simulink model "model_0318"  (R2025b)
settings: Solver=ode4  StartTime=0.0  StopTime=10  FixedStep=1e-4  RelTol=1e-3
undefined symbols (not defined in the file or in its folder): dspblkCoreblockFVToolHelper, gcbh
libraries: simulink x9, dspfdesign x3, dspstat3 x2

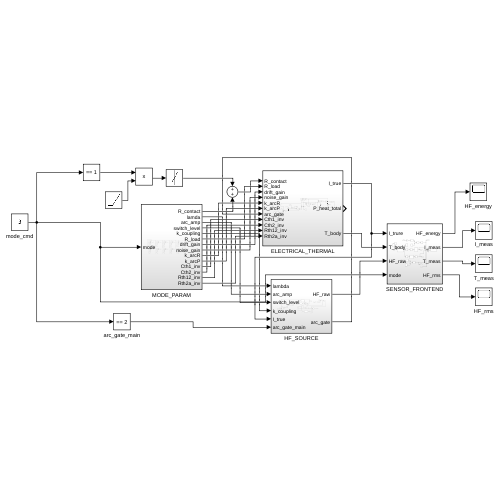
[thumbnail: Simulink's stored preview of the top-level diagram]
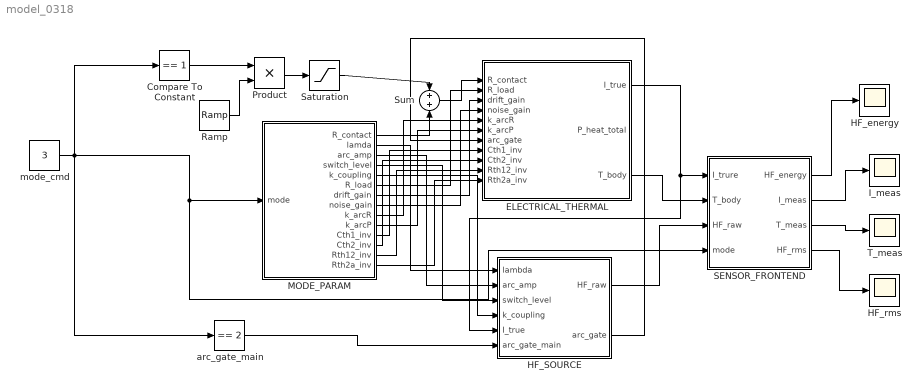
== system model_0318 ==
  Compare To Constant : simulink/Logic and Bit Operations/Compare To Constant  relop===  const=1  OutDataTypeStr=boolean
  ELECTRICAL_THERMAL : Subsystem
  HF_SOURCE : Subsystem
  HF_energy : Scope
      settings: ActiveDisplayYMinimum=-0.0012745703984799416  ActiveDisplayYMaximum=0.011471133695894987
  HF_rms : Scope
      settings: ActiveDisplayYMinimum=-0.0022642888342853068  ActiveDisplayYMaximum=0.020378601958750724  DataLoggingVariableName=ScopeData3
  I_meas : Scope
      settings: ActiveDisplayYMinimum=-209.09631630294618  ActiveDisplayYMaximum=207.20339945692962
  MODE_PARAM : Subsystem
  Product : Product
  Ramp : simulink/Sources/Ramp  slope=0.002  start=0  InitialOutput=0
  SENSOR_FRONTEND : Subsystem
  Saturation : Saturate  UpperLimit=0.05  LowerLimit=0
  Sum : Sum
  T_meas : Scope
      settings: ActiveDisplayYMinimum=19.005455597500632  ActiveDisplayYMaximum=28.950899622494315  DataLoggingVariableName=ScopeData2
  arc_gate_main : simulink/Logic and Bit Operations/Compare To Constant  relop===  const=2  OutDataTypeStr=boolean
  mode_cmd : Constant  Value=3
  wires:
  ELECTRICAL_THERMAL/1(I_true) -> HF_SOURCE/5(I_true), SENSOR_FRONTEND/1(I_trure)
  mode_cmd/1 -> arc_gate_main/1, SENSOR_FRONTEND/4(mode), MODE_PARAM/1(mode), Compare To Constant/1
  Compare To Constant/1 -> Product/1
  Ramp/1 -> Product/2
  Product/1 -> Saturation/1
  Saturation/1 -> Sum/1
  MODE_PARAM/1(R_contact) -> Sum/2
  Sum/1 -> ELECTRICAL_THERMAL/1(R_contact)
  SENSOR_FRONTEND/2(I_meas) -> I_meas/1
  SENSOR_FRONTEND/3(T_meas) -> T_meas/1
  SENSOR_FRONTEND/1(HF_energy) -> HF_energy/1
  SENSOR_FRONTEND/4(HF_rms) -> HF_rms/1
  MODE_PARAM/6(R_load) -> ELECTRICAL_THERMAL/2(R_load)
  MODE_PARAM/7(drift_gain) -> ELECTRICAL_THERMAL/3(drift_gain)
  MODE_PARAM/8(noise_gain) -> ELECTRICAL_THERMAL/4(noise_gain)
  MODE_PARAM/9(k_arcR) -> ELECTRICAL_THERMAL/5(k_arcR)
  MODE_PARAM/10(k_arcP) -> ELECTRICAL_THERMAL/6(k_arcP)
  MODE_PARAM/11(Cth1_inv) -> ELECTRICAL_THERMAL/8(Cth1_inv)
  MODE_PARAM/12(Cth2_inv) -> ELECTRICAL_THERMAL/9(Cth2_inv)
  MODE_PARAM/13(Rth12_inv) -> ELECTRICAL_THERMAL/10(Rth12_inv)
  MODE_PARAM/14(Rth2a_inv) -> ELECTRICAL_THERMAL/11(Rth2a_inv)
  MODE_PARAM/3(arc_amp) -> HF_SOURCE/2(arc_amp)
  MODE_PARAM/2(lamda) -> HF_SOURCE/1(lambda)
  MODE_PARAM/5(k_coupling) -> HF_SOURCE/4(k_coupling)
  MODE_PARAM/4(switch_level) -> HF_SOURCE/3(switch_level)
  HF_SOURCE/2(arc_gate) -> ELECTRICAL_THERMAL/7(arc_gate)
  HF_SOURCE/1(HF_raw) -> SENSOR_FRONTEND/3(HF_raw)
  ELECTRICAL_THERMAL/3(T_body) -> SENSOR_FRONTEND/2(T_body)
  arc_gate_main/1 -> HF_SOURCE/6(arc_gate_main)

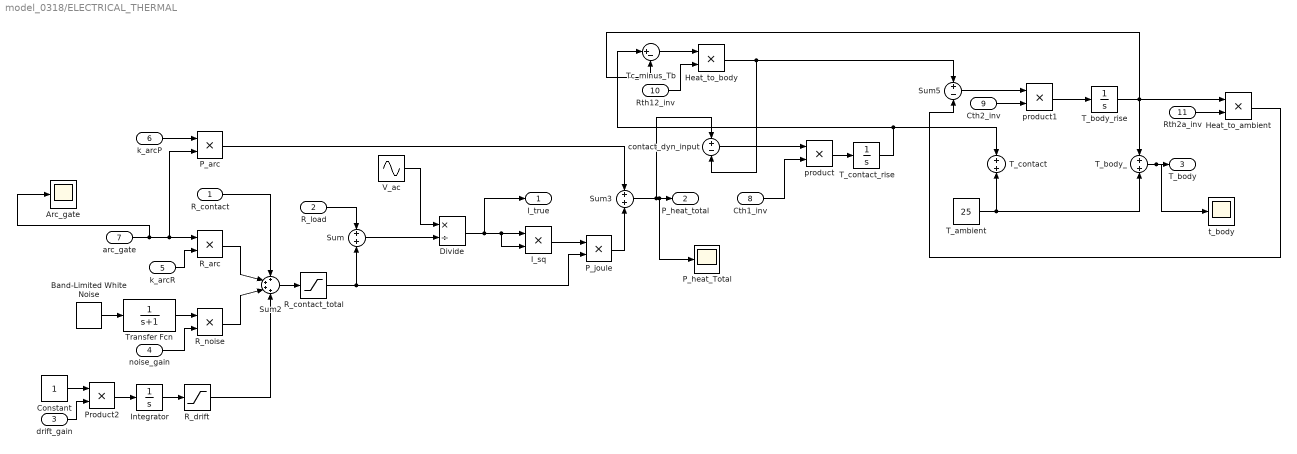
== system model_0318/ELECTRICAL_THERMAL ==
  R_contact : Inport
  R_load : Inport  Port=2
  drift_gain : Inport  Port=3
  noise_gain : Inport  Port=4
  k_arcR : Inport  Port=5
  k_arcP : Inport  Port=6
  arc_gate : Inport  Port=7
  Cth1_inv : Inport  Port=8
  Cth2_inv : Inport  Port=9
  Rth12_inv : Inport  Port=10
  Rth2a_inv : Inport  Port=11
  Arc_gate : Scope
      settings: ActiveDisplayYMinimum=-1  ActiveDisplayYMaximum=1  DataLoggingVariableName=ScopeData5
  Band-Limited White Noise : simulink/Sources/Band-Limited White Noise  Cov=1e-4  Ts=1e-4  seed=11
  Constant : Constant
  Divide : Product  Inputs=*/
  Heat_to_ambient : Product
  Heat_to_body : Product
  I_sq : Product
  Integrator : Integrator
  P_arc : Product
  P_heat_Total : Scope
      settings: ActiveDisplayYMinimum=-108.37902275446248  ActiveDisplayYMaximum=975.41120479016263  DataLoggingVariableName=ScopeData4
  P_joule : Product
  Product2 : Product
  R_arc : Product
  R_contact_total : Saturate  UpperLimit=1  LowerLimit=0.001
  R_drift : Saturate
  R_noise : Product
  Sum : Sum
  Sum2 : Sum  Inputs=++++
  Sum3 : Sum
  Sum5 : Sum  Inputs=+-
  T_ambient : Constant  Value=25
  T_body_ : Sum
  T_body_rise : Integrator
  T_contact : Sum
  T_contact_rise : Integrator
  Tc_minus_Tb : Sum  Inputs=|+-
  Transfer Fcn : TransferFcn  Denominator=[1 1]
  V_ac : Sin  Amplitude=311  Frequency=2*pi*60  SampleTime=1e-4
  contact_dyn_input : Sum  Inputs=+-
  product : Product
  product1 : Product
  t_body : Scope
      settings: ActiveDisplayYMinimum=14.417043129702609  ActiveDisplayYMaximum=120.24661183267655  DataLoggingVariableName=ScopeData7
  I_true : Outport
  P_heat_total : Outport  Port=2
  T_body : Outport  Port=3
  wires:
  R_load/1 -> Sum/1
  Sum/1 -> Divide/2
  V_ac/1 -> Divide/1
  Divide/1 -> I_sq/2, I_sq/1, I_true/1
  I_sq/1 -> P_joule/1
  P_joule/1 -> Sum3/2
  Band-Limited White Noise/1 -> Transfer Fcn/1
  Constant/1 -> Product2/1
  drift_gain/1 -> Product2/2
  Product2/1 -> Integrator/1
  Integrator/1 -> R_drift/1
  Transfer Fcn/1 -> R_noise/1
  noise_gain/1 -> R_noise/2
  arc_gate/1 -> Arc_gate/1, P_arc/2, R_arc/1
  k_arcR/1 -> R_arc/2
  R_contact/1 -> Sum2/1
  R_arc/1 -> Sum2/2
  R_noise/1 -> Sum2/3
  R_drift/1 -> Sum2/4
  Sum2/1 -> R_contact_total/1
  R_contact_total/1 -> P_joule/2, Sum/2
  k_arcP/1 -> P_arc/1
  P_arc/1 -> Sum3/1
  Sum3/1 -> contact_dyn_input/1, P_heat_Total/1, P_heat_total/1
  Tc_minus_Tb/1 -> Heat_to_body/1
  Heat_to_body/1 -> contact_dyn_input/2, Sum5/1
  Cth1_inv/1 -> product/2
  contact_dyn_input/1 -> product/1
  product/1 -> T_contact_rise/1
  T_contact_rise/1 -> T_contact/1, Tc_minus_Tb/1
  Sum5/1 -> product1/1
  Cth2_inv/1 -> product1/2
  product1/1 -> T_body_rise/1
  T_body_rise/1 -> T_body_/1, Heat_to_ambient/1, Tc_minus_Tb/2
  T_ambient/1 -> T_contact/2, T_body_/2
  Rth12_inv/1 -> Heat_to_body/2
  Rth2a_inv/1 -> Heat_to_ambient/2
  Heat_to_ambient/1 -> Sum5/2
  T_body_/1 -> t_body/1, T_body/1

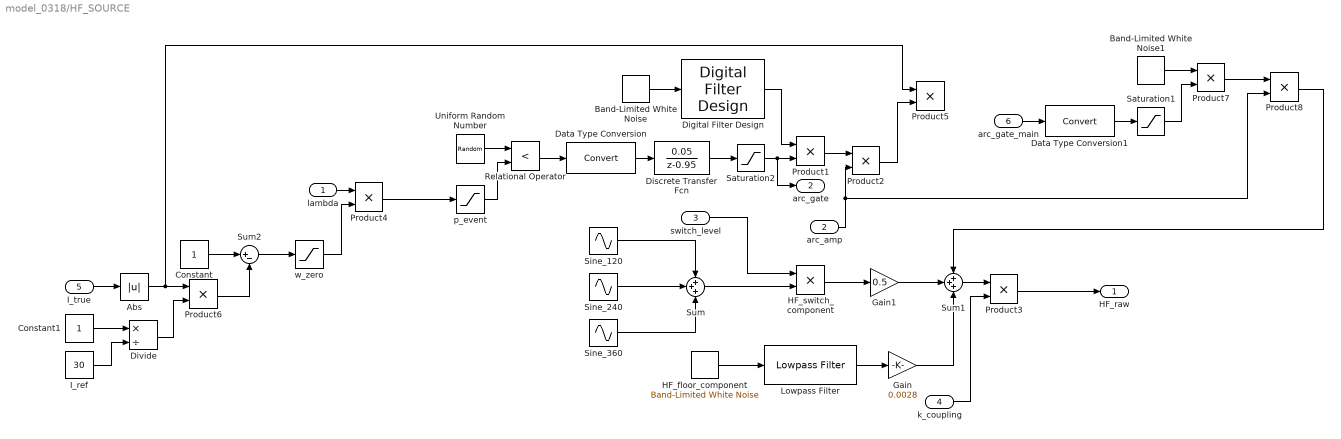
== system model_0318/HF_SOURCE ==
  lambda : Inport
  arc_amp : Inport  Port=2
  switch_level : Inport  Port=3
  k_coupling : Inport  Port=4
  I_true : Inport  Port=5
  arc_gate_main : Inport  Port=6
  Abs : Abs  SaturateOnIntegerOverflow=off
  Band-Limited White Noise : simulink/Sources/Band-Limited White Noise  Cov=1  Ts=1e-4  seed=0
  Band-Limited White Noise1 : simulink/Sources/Band-Limited White Noise  Cov=1  Ts=1e-4  seed=0
  Constant : Constant
  Constant1 : Constant
  Data Type Conversion : DataTypeConversion  SaturateOnIntegerOverflow=off  RndMeth=Floor
  Data Type Conversion1 : DataTypeConversion  SaturateOnIntegerOverflow=off  RndMeth=Floor
  Digital Filter Design : dspfdesign/Digital Filter Design  mwdsp_browser_bugfix_var=off
  Discrete Transfer Fcn : DiscreteTransferFcn  LoadFcn=dspblkCoreblockFVToolHelper(gcbh,'load');  Numerator=[0.05]  Denominator=[1 -0.95]
      settings: CopyFcn=dspblkCoreblockFVToolHelper(gcbh,'copy');  DeleteFcn=dspblkCoreblockFVToolHelper(gcbh,'close');  ModelCloseFcn=dspblkCoreblockFVToolHelper(gcbh,'close');  PreSaveFcn=dspblkCoreblockFVToolHelper(gcbh,'presave');  PostSaveFcn=dspblkCoreblockFVToolHelper(gcbh,'postsave');  CloseFcn=dspblkCoreblockFVToolHelper(gcbh,'close');
  Divide : Product  Inputs=*/
  Gain : Gain  Gain=0.0028
  Gain1 : Gain  Gain=0.5
  HF_floor_component : simulink/Sources/Band-Limited White Noise  Cov=5e-3  Ts=1e-4  seed=31
  HF_switch_component : Product
  I_ref : Constant  Value=30
  Lowpass Filter : dspfdesign/Lowpass Filter  FilterType=FIR  DesignForMinimumOrder=on  FilterOrder=50  PassbandFrequency=0.04  StopbandFrequency=0.08  PassbandRipple=0.1  StopbandAttenuation=80  SampleRateMode=Use normalized frequency (0 to 1)  SampleRate=44100  SimulateUsing=Interpreted execution  roundingMode=Floor  coeffsDataTypeStr=fixdt(1,16)
  Product{1..8} (8 alike) : Product
  Relational Operator : RelationalOperator  Operator=<  OutDataTypeStr=boolean  RndMeth=Simplest  InputSameDT=off
  Saturation1 : Saturate  UpperLimit=1  LowerLimit=0
  Saturation2 : Saturate  UpperLimit=1  LowerLimit=0
  Sine_120 : Sin  SineType=Sample based  Amplitude=0.2  Frequency=2*pi*120  Samples=83  SampleTime=1e-4
  Sine_240 : Sin  SineType=Sample based  Amplitude=0.15  Frequency=2*pi*240  Samples=42  SampleTime=1e-4
  Sine_360 : Sin  SineType=Sample based  Amplitude=0.1  Frequency=2*pi*360  Samples=28  SampleTime=1e-4
  Sum : Sum  Inputs=+++
  Sum1 : Sum  Inputs=+++
  Sum2 : Sum  Inputs=|+-
  Uniform Random Number : UniformRandomNumber  Minimum=0  Seed=21  SampleTime=1e-4
  p_event : Saturate  UpperLimit=1  LowerLimit=0
  w_zero : Saturate  UpperLimit=1  LowerLimit=0
  HF_raw : Outport
  arc_gate : Outport  Port=2
  wires:
  Sine_240/1 -> Sum/2
  Sine_120/1 -> Sum/1
  Sine_360/1 -> Sum/3
  Sum/1 -> HF_switch_component/2
  switch_level/1 -> HF_switch_component/1
  Product4/1 -> p_event/1
  Uniform Random Number/1 -> Relational Operator/1
  p_event/1 -> Relational Operator/2
  k_coupling/1 -> Product3/2
  Product1/1 -> Product2/1
  I_true/1 -> Abs/1
  Abs/1 -> Product5/1, Product6/1
  lambda/1 -> Product4/1
  w_zero/1 -> Product4/2
  Constant/1 -> Sum2/1
  Product6/1 -> Sum2/2
  Sum2/1 -> w_zero/1
  Discrete Transfer Fcn/1 -> Saturation2/1
  Saturation2/1 -> arc_gate/1, Product1/2
  I_ref/1 -> Divide/2
  Constant1/1 -> Divide/1
  Divide/1 -> Product6/2
  Product2/1 -> Product5/2
  Band-Limited White Noise/1 -> Digital Filter Design/1
  Digital Filter Design/1 -> Product1/1
  HF_floor_component/1 -> Lowpass Filter/1
  Data Type Conversion/1 -> Discrete Transfer Fcn/1
  Relational Operator/1 -> Data Type Conversion/1
  Sum1/1 -> Product3/1
  Lowpass Filter/1 -> Gain/1
  Gain/1 -> Sum1/3
  HF_switch_component/1 -> Gain1/1
  Gain1/1 -> Sum1/2
  Band-Limited White Noise1/1 -> Product7/1
  Product7/1 -> Product8/1
  arc_amp/1 -> Product8/2, Product2/2
  Product8/1 -> Sum1/1
  Product3/1 -> HF_raw/1
  Saturation1/1 -> Product7/2
  arc_gate_main/1 -> Data Type Conversion1/1
  Data Type Conversion1/1 -> Saturation1/1

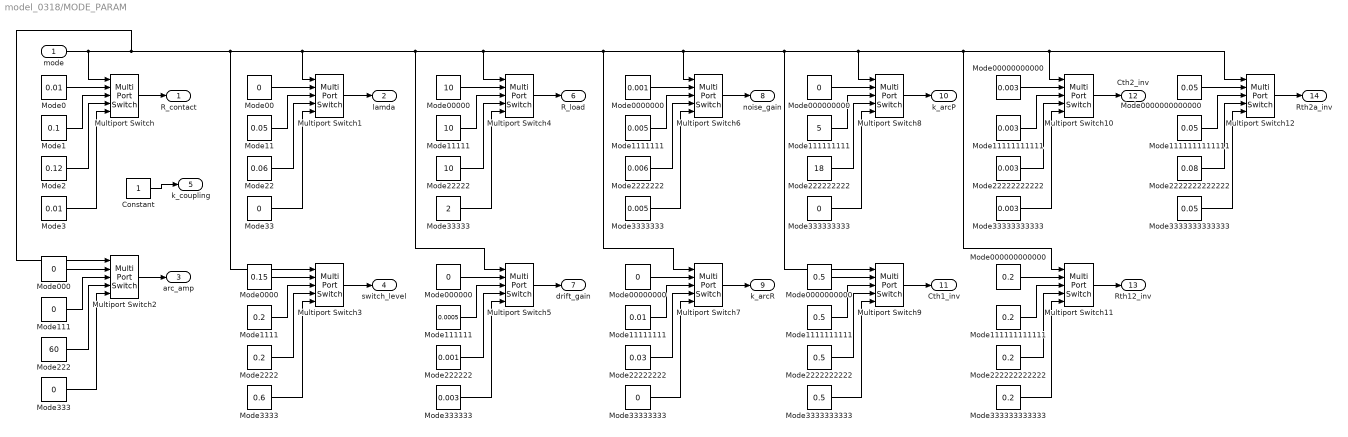
== system model_0318/MODE_PARAM ==
  mode : Inport
  Constant : Constant
  Mode0 : Constant  Value=0.01
  Mode00 : Constant  Value=0
  Mode000 : Constant  Value=0
  Mode0000 : Constant  Value=0.15
  Mode00000 : Constant  Value=10
  Mode000000 : Constant  Value=0
  Mode0000000 : Constant  Value=0.001
  Mode00000000 : Constant  Value=0
  Mode000000000 : Constant  Value=0
  Mode0000000000 : Constant  Value=0.5
  Mode00000000000 : Constant  Value=0.003
  Mode000000000000 : Constant  Value=0.2
  Mode0000000000000 : Constant  Value=0.05
  Mode1 : Constant  Value=0.1
  Mode11 : Constant  Value=0.05
  Mode{33,111,333,33333333,333333333} (5 alike) : Constant  Value=0
  Mode{1111,2222,111111111111,222222222222,333333333333} (5 alike) : Constant  Value=0.2
  Mode11111 : Constant  Value=10
  Mode111111 : Constant  Value=0.0005
  Mode1111111 : Constant  Value=0.005
  Mode11111111 : Constant  Value=0.01
  Mode111111111 : Constant  Value=5
  Mode1111111111 : Constant  Value=0.5
  Mode{333333,11111111111,22222222222,33333333333} (4 alike) : Constant  Value=0.003
  Mode1111111111111 : Constant  Value=0.05
  Mode2 : Constant  Value=0.12
  Mode22 : Constant  Value=0.06
  Mode222 : Constant  Value=60
  Mode22222 : Constant  Value=10
  Mode222222 : Constant  Value=0.001
  Mode2222222 : Constant  Value=0.006
  Mode22222222 : Constant  Value=0.03
  Mode222222222 : Constant  Value=18
  Mode2222222222 : Constant  Value=0.5
  Mode2222222222222 : Constant  Value=0.08
  Mode3 : Constant  Value=0.01
  Mode3333 : Constant  Value=0.6
  Mode33333 : Constant  Value=2
  Mode3333333 : Constant  Value=0.005
  Mode3333333333 : Constant  Value=0.5
  Mode3333333333333 : Constant  Value=0.05
  Multiport Switch{,1..12} (13 alike) : MultiPortSwitch  DataPortOrder=Zero-based contiguous  Inputs=4  zeroidx=on  SaturateOnIntegerOverflow=off  InputSameDT=off
  R_contact : Outport
  lamda : Outport  Port=2
  arc_amp : Outport  Port=3
  switch_level : Outport  Port=4
  k_coupling : Outport  Port=5
  R_load : Outport  Port=6
  drift_gain : Outport  Port=7
  noise_gain : Outport  Port=8
  k_arcR : Outport  Port=9
  k_arcP : Outport  Port=10
  Cth1_inv : Outport  Port=11
  Cth2_inv : Outport  Port=12
  Rth12_inv : Outport  Port=13
  Rth2a_inv : Outport  Port=14
  wires:
  Mode0/1 -> Multiport Switch/2
  Mode1/1 -> Multiport Switch/3
  Mode2/1 -> Multiport Switch/4
  Mode3/1 -> Multiport Switch/5
  mode/1 -> Multiport Switch2/1, Multiport Switch5/1, Multiport Switch7/1, Multiport Switch6/1, Multiport Switch11/1, Multiport Switch10/1, Multiport Switch12/1, Multiport Switch8/1, Multiport Switch9/1, Multiport Switch4/1, Multiport Switch1/1, Multiport Switch3/1, Multiport Switch/1
  Multiport Switch/1 -> R_contact/1
  Multiport Switch1/1 -> lamda/1
  Mode33/1 -> Multiport Switch1/5
  Mode22/1 -> Multiport Switch1/4
  Mode11/1 -> Multiport Switch1/3
  Mode00/1 -> Multiport Switch1/2
  Mode000/1 -> Multiport Switch2/2
  Mode111/1 -> Multiport Switch2/3
  Mode222/1 -> Multiport Switch2/4
  Mode333/1 -> Multiport Switch2/5
  Multiport Switch2/1 -> arc_amp/1
  Multiport Switch3/1 -> switch_level/1
  Mode3333/1 -> Multiport Switch3/5
  Mode2222/1 -> Multiport Switch3/4
  Mode1111/1 -> Multiport Switch3/3
  Mode0000/1 -> Multiport Switch3/2
  Constant/1 -> k_coupling/1
  Mode00000/1 -> Multiport Switch4/2
  Mode11111/1 -> Multiport Switch4/3
  Mode22222/1 -> Multiport Switch4/4
  Mode33333/1 -> Multiport Switch4/5
  Multiport Switch4/1 -> R_load/1
  Multiport Switch5/1 -> drift_gain/1
  Mode333333/1 -> Multiport Switch5/5
  Mode222222/1 -> Multiport Switch5/4
  Mode111111/1 -> Multiport Switch5/3
  Mode000000/1 -> Multiport Switch5/2
  Mode0000000/1 -> Multiport Switch6/2
  Mode1111111/1 -> Multiport Switch6/3
  Mode2222222/1 -> Multiport Switch6/4
  Mode3333333/1 -> Multiport Switch6/5
  Multiport Switch6/1 -> noise_gain/1
  Multiport Switch7/1 -> k_arcR/1
  Mode33333333/1 -> Multiport Switch7/5
  Mode22222222/1 -> Multiport Switch7/4
  Mode11111111/1 -> Multiport Switch7/3
  Mode00000000/1 -> Multiport Switch7/2
  Mode000000000/1 -> Multiport Switch8/2
  Mode111111111/1 -> Multiport Switch8/3
  Mode222222222/1 -> Multiport Switch8/4
  Mode333333333/1 -> Multiport Switch8/5
  Multiport Switch8/1 -> k_arcP/1
  Multiport Switch9/1 -> Cth1_inv/1
  Mode3333333333/1 -> Multiport Switch9/5
  Mode2222222222/1 -> Multiport Switch9/4
  Mode1111111111/1 -> Multiport Switch9/3
  Mode0000000000/1 -> Multiport Switch9/2
  Multiport Switch12/1 -> Rth2a_inv/1
  Mode3333333333333/1 -> Multiport Switch12/5
  Mode2222222222222/1 -> Multiport Switch12/4
  Mode1111111111111/1 -> Multiport Switch12/3
  Mode0000000000000/1 -> Multiport Switch12/2
  Mode000000000000/1 -> Multiport Switch11/2
  Mode111111111111/1 -> Multiport Switch11/3
  Mode222222222222/1 -> Multiport Switch11/4
  Mode333333333333/1 -> Multiport Switch11/5
  Multiport Switch11/1 -> Rth12_inv/1
  Multiport Switch10/1 -> Cth2_inv/1
  Mode33333333333/1 -> Multiport Switch10/5
  Mode22222222222/1 -> Multiport Switch10/4
  Mode11111111111/1 -> Multiport Switch10/3
  Mode00000000000/1 -> Multiport Switch10/2

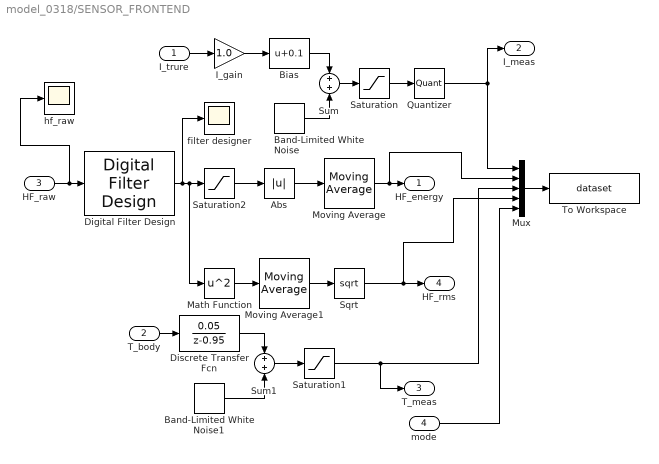
== system model_0318/SENSOR_FRONTEND ==
  I_trure : Inport
  T_body : Inport  Port=2
  HF_raw : Inport  Port=3
  mode : Inport  Port=4
  Abs : Abs  SaturateOnIntegerOverflow=off
  Band-Limited White Noise : simulink/Sources/Band-Limited White Noise  Cov=1e-5  Ts=1e-4  seed=41
  Band-Limited White Noise1 : simulink/Sources/Band-Limited White Noise  Cov=1e-6  Ts=1e-4  seed=51
  Bias : Bias  Bias=0.1  SaturateOnIntegerOverflow=off
  Digital Filter Design : dspfdesign/Digital Filter Design  mwdsp_browser_bugfix_var=off
  Discrete Transfer Fcn : DiscreteTransferFcn  LoadFcn=dspblkCoreblockFVToolHelper(gcbh,'load');  Numerator=[0.05]  Denominator=[1 -0.95]
      settings: CopyFcn=dspblkCoreblockFVToolHelper(gcbh,'copy');  DeleteFcn=dspblkCoreblockFVToolHelper(gcbh,'close');  ModelCloseFcn=dspblkCoreblockFVToolHelper(gcbh,'close');  PreSaveFcn=dspblkCoreblockFVToolHelper(gcbh,'presave');  PostSaveFcn=dspblkCoreblockFVToolHelper(gcbh,'postsave');  CloseFcn=dspblkCoreblockFVToolHelper(gcbh,'close');
  I_gain : Gain  Gain=1.0
  Math Function : Math  Operator=square
  Moving Average : dspstat3/Moving Average  Method=Sliding window  ForgettingFactorPort=off  SpecifyWindowLength=on  WindowLength=100  OverlapLength=99  AllowArbitraryInputLength=off  ForgettingFactor=0.9  SimulateUsing=Interpreted execution
  Moving Average1 : dspstat3/Moving Average  Method=Sliding window  ForgettingFactorPort=off  SpecifyWindowLength=on  WindowLength=20  OverlapLength=19  AllowArbitraryInputLength=off  ForgettingFactor=0.9  SimulateUsing=Interpreted execution
  Mux : Mux  Inputs=5
  Quantizer : Quantizer  QuantizationInterval=0.1
  Saturation : Saturate  UpperLimit=200  LowerLimit=-200
  Saturation1 : Saturate  UpperLimit=120  LowerLimit=20
  Saturation2 : Saturate  UpperLimit=5  LowerLimit=-5
  Sqrt : Sqrt
  Sum : Sum
  Sum1 : Sum
  To Workspace : ToWorkspace  VariableName=dataset  SampleTime=-1
  filter designer : Scope
      settings: ActiveDisplayYMinimum=-0.035382118179874689  ActiveDisplayYMaximum=0.025626438107198959  DataLoggingVariableName=ScopeData6
  hf_raw : Scope
      settings: ActiveDisplayYMinimum=-0.17521192271608907  ActiveDisplayYMaximum=0.17555885867388121  DataLoggingVariableName=ScopeData8
  HF_energy : Outport
  I_meas : Outport  Port=2
  T_meas : Outport  Port=3
  HF_rms : Outport  Port=4
  wires:
  Abs/1 -> Moving Average/1
  Moving Average/1 -> Mux/2, HF_energy/1
  I_trure/1 -> I_gain/1
  Band-Limited White Noise/1 -> Sum/2
  Band-Limited White Noise1/1 -> Sum1/2
  Mux/1 -> To Workspace/1
  HF_raw/1 -> hf_raw/1, Digital Filter Design/1
  Saturation/1 -> Quantizer/1
  I_gain/1 -> Bias/1
  Bias/1 -> Sum/1
  Sum/1 -> Saturation/1
  Quantizer/1 -> I_meas/1, Mux/1
  Saturation1/1 -> T_meas/1, Mux/3
  Sum1/1 -> Saturation1/1
  Moving Average1/1 -> Sqrt/1
  Saturation2/1 -> Abs/1
  Sqrt/1 -> Mux/4, HF_rms/1
  Math Function/1 -> Moving Average1/1
  T_body/1 -> Discrete Transfer Fcn/1
  Discrete Transfer Fcn/1 -> Sum1/1
  mode/1 -> Mux/5
  Digital Filter Design/1 -> filter designer/1, Math Function/1, Saturation2/1
